simulink model "Vehicle_Model_14DOF"  (R2020a)
settings: Solver=ode23s  StartTime=0.0  StopTime=8  RelTol=1e-2  EnableMultiTasking=on
model workspace (MAT data in the model file):
  Csfl = 100
  Csfr = 100
  Csrl = 100
  Csrr = 100
  Hp = 0.35
  Ksfl = 100
  Ksfr = 100
  Ksrl = 100
  Ksrr = 100
undefined symbols (not defined in the file): sigbuilder_block
libraries: simulink_extras x6, simulink x1
(part 3 of 3)

== matlab function Vehicle_Model_14DOF/Full vehicle 14 D.O.F /Vehicle Handling model 7D.O.F /Yaw axis d,o,f /Sigma  moment Yaw axis ==
  data: A_O input; A_i input; Yaw output; Fxfl input; Fyfl input; Fxfr input; Fyfr input; Fxrl input; Fyrl input; Fxrr input; Fyrr input; Mzfl input; Mzfr input; Mzrl input; Mzrr input; wf input; wr input; a input; b input
function Yaw = fcn(A_O,A_i,Fxfl,Fyfl,Fxfr,Fyfr,Fxrl,Fyrl,Fxrr,Fyrr,Mzfl,Mzfr,Mzrl,Mzrr,wf,wr,a,b)

Yaw =(-(wf./2).*Fxfl.*cos(A_O))+((wf./2).*Fxfr.*cos(A_i))-((wr./2).*Fxrl)+((wr./2).*Fxrr)+((wf./2).*Fyfl.*sin(A_O))-((wf./2).*Fyfr.*sin(A_i))+(a.*Fxfl.*sin(A_O))+(a.*Fyfl.*cos(A_O))+(a.*Fxfr.*sin(A_i))+(a.*Fyfr.*cos(A_i))-(b.*Fyrl)-(b.*Fyrr)+(Mzfl)+(Mzfr)+(Mzrl)+(Mzrr);

== matlab function Vehicle_Model_14DOF/Full vehicle 14 D.O.F /Tiremodel/Tire front right/Fx/MATLAB Function ==
  data: ffz input; Fx output; xx input
function Fx = fcn(ffz,xx)

%xx is the slip ratio -- expressed as fraction
D=2.776
C=1.6099
B=14.3014
E=1.0224
sv=0.1221
sh=0
Fx = D.* ffz .*sin(C.* atan((B.*(xx+sh*ffz))- E*(B.* (xx+sh*ffz)- atan(B.*(xx+sh*ffz))))) ;

== matlab function Vehicle_Model_14DOF/Full vehicle 14 D.O.F /Vehicle Handling model 7D.O.F /Longtudinal axis D.O.F /MATLAB Function ==
  data: A_o input; A_i input; AX output; Fxfl input; Fyfl input; Fxfr input; Fyfr input; Fxrl input; Fxrr input; Vx input; Ro input; Ar input; Cd input
function AX = fcn(A_o,A_i,Fxfl,Fyfl,Fxfr,Fyfr,Fxrl,Fxrr, Vx, Ro, Ar, Cd)

AX = Fxfl.*cos(A_o)-Fyfl.*sin(A_o)+Fxfr.*cos(A_i)-Fyfr.*sin(A_i)+Fxrr+Fxrl - 1/2 .* Vx.^2 .* Ro .* Ar .* Cd - 70;

== matlab function Vehicle_Model_14DOF/Full vehicle 14 D.O.F /Vehicle Handling model 7D.O.F /Lateral Axis D.o.f /MATLAB Function ==
  data: A_o input; A_i input; AY output; Fyfl input; Fxfl input; Fyfr input; Fxfr input; Fyrl input; Fyrr input
function AY = fcn(A_o,A_i,Fyfl,Fxfl,Fyfr,Fxfr,Fyrl,Fyrr)

AY = Fyfl.*cos(A_o)+Fxfl.*sin(A_o)+Fyfr.*cos(A_i)+Fxfr.*sin(A_i)+Fyrl+Fyrr;

== matlab function Vehicle_Model_14DOF/Full vehicle 14 D.O.F /Vehicle Handling model 7D.O.F /Powertrain /MATLAB Function4 ==
  data: T input; Fx input; RPM input; m output; Rw input
function m = fcn(T, Fx, RPM, Rw)
if (RPM > 15100)
    m = Fx * Rw;
else
    m=T;
end
end

== matlab function Vehicle_Model_14DOF/Full vehicle 14 D.O.F /Tiremodel/Tire front left/Fx/MATLAB Function ==
  data: ffz input; Fx output; xx input
function Fx = fcn(ffz,xx)

%xx is the slip ratio -- expressed as fraction
D=2.776
C=1.6099
B=14.3014
E=1.0224
sv=0.1221
sh=0
Fx = D.* ffz .*sin(C.* atan((B.*(xx+sh*ffz))- E*(B.* (xx+sh*ffz)- atan(B.*(xx+sh*ffz))))) ;

== matlab function Vehicle_Model_14DOF/Full vehicle 14 D.O.F /Vehicle Handling model 7D.O.F /Powertrain /MATLAB Function5 ==
  data: T input; Fx input; RPM input; m output; Rw input
function m = fcn(T, Fx, RPM, Rw)
if (RPM > 15100)
    m = Fx * Rw;
else
    m=T;
end
end

== matlab function Vehicle_Model_14DOF/Full vehicle 14 D.O.F /Tiremodel/LCO width 6 psi 14/Fx/MATLAB Function ==
  data: ffz input; Fx output; xx input
function Fx = fcn(ffz,xx)

%xx is the slip ratio -- expressed as fraction
D= 12.3158
C=0.2162
B=12.9458 
E=1.0917


sv=0
sh=0
Fx = D.* ffz .*sin(C.* atan((B.*(xx+sh*ffz))- E*(B.* (xx+sh*ffz)- atan(B.*(xx+sh*ffz))))) + sv*ffz;

== matlab function Vehicle_Model_14DOF/Full vehicle 14 D.O.F /Tiremodel/Tire front left/fy/MATLAB Function ==
  data: ffz input; Fx output; xx input
function Fx = fcn(ffz,xx)

%xx is the slip ratio -- expressed as fraction
D = -2.8334
C =  1.5184
B =    0.2461
E =   0.4953


Fx = D.* ffz .*sin(C.* atan((B.*(xx))- E*(B.* (xx)- atan(B.*(xx))))) ;

== matlab function Vehicle_Model_14DOF/Full vehicle 14 D.O.F /Tiremodel/LCO width 6 psi 14/fy/MATLAB Function ==
  data: ffz input; Fx output; xx input
function Fx = fcn(ffz,xx)

%xx is the slip ratio -- expressed as fraction
D=-2.4199
C=3.6531
B=0.0586
E=3.1915





Fx = D.* ffz .*sin(C.* atan((B.*(xx))- E*(B.* (xx)- atan(B.*(xx))))) ;

== matlab function Vehicle_Model_14DOF/Full vehicle 14 D.O.F /Tiremodel/LCO width 6 psi 14/fy1/MZ/MATLAB Function ==
  data: ffz input; Fx output; xx input
function Fx = fcn(ffz,xx)

%xx is the slip ratio -- expressed as fraction
D=-14.1402
C=-0.0029
B=1.0476
E=1.1218



Fx = D.* ffz .*sin(C.* atan((B.*(xx))- E*(B.* (xx)- atan(B.*(xx))))) ;

== matlab function Vehicle_Model_14DOF/Full vehicle 14 D.O.F /Tiremodel/R25b width 7 psi 14/Fx/MATLAB Function ==
  data: ffz input; Fx output; xx input
function Fx = fcn(ffz,xx)

%xx is the slip ratio -- expressed as fraction
D=2.3835
C=1.1725
B=14.4401
E=0.1925

sv=0
sh=0
Fx = D.* ffz .*sin(C.* atan((B.*(xx+sh*ffz))- E*(B.* (xx+sh*ffz)- atan(B.*(xx+sh*ffz))))) + sv*ffz;

== matlab function Vehicle_Model_14DOF/Full vehicle 14 D.O.F /Tiremodel/R25b width 7 psi 14/fy/MATLAB Function ==
  data: ffz input; Fx output; xx input
function Fx = fcn(ffz,xx)

%xx is the slip ratio -- expressed as fraction
D= -2.5960
C= 1.6785    
B= 0.1612    
E= 1.3667



Fx = D.* ffz .*sin(C.* atan((B.*(xx))- E*(B.* (xx)- atan(B.*(xx))))) ;

== matlab function Vehicle_Model_14DOF/Full vehicle 14 D.O.F /Tiremodel/R25b width 7 psi 14/fy1/MZ/MATLAB Function ==
  data: ffz input; Fx output; xx input
function Fx = fcn(ffz,xx)

%xx is the slip ratio -- expressed as fraction
D = -0.8015
C = -0.0512
B = 0.8235
E = 1.1950



Fx = D.* ffz .*sin(C.* atan((B.*(xx))- E*(B.* (xx)- atan(B.*(xx))))) ;

== matlab function Vehicle_Model_14DOF/Full vehicle 14 D.O.F /Tiremodel/R25b width 6 psi 14/Fx/MATLAB Function ==
  data: ffz input; Fx output; xx input
function Fx = fcn(ffz,xx)

%xx is the slip ratio -- expressed as fraction
D= 2.4699    
C=0.8676   
B=15.9036    
E=0.1161

sv=0
sh=0
Fx = D.* ffz .*sin(C.* atan((B.*(xx+sh*ffz))- E*(B.* (xx+sh*ffz)- atan(B.*(xx+sh*ffz))))) + sv*ffz;

== matlab function Vehicle_Model_14DOF/Full vehicle 14 D.O.F /Tiremodel/R25b width 6 psi 14/fy/MATLAB Function ==
  data: ffz input; Fx output; xx input
function Fx = fcn(ffz,xx)

%xx is the slip ratio -- expressed as fraction
D= -2.4262 
C= 38.3467
B= 0.0066
E= 230



Fx = D.* ffz .*sin(C.* atan((B.*(xx))- E*(B.* (xx)- atan(B.*(xx))))) ;

== matlab function Vehicle_Model_14DOF/Full vehicle 14 D.O.F /Tiremodel/R25b width 6 psi 14/fy1/MZ/MATLAB Function ==
  data: ffz input; Fx output; xx input
function Fx = fcn(ffz,xx)

%xx is the slip ratio -- expressed as fraction
D = -0.8415
C = -0.0512
B = 0.8235
E = 1.1959




Fx = D.* ffz .*sin(C.* atan((B.*(xx))- E*(B.* (xx)- atan(B.*(xx))))) ;

== matlab function Vehicle_Model_14DOF/Full vehicle 14 D.O.F /Tiremodel/R25b width 7 psi 10/Fx/MATLAB Function ==
  data: ffz input; Fx output; xx input
function Fx = fcn(ffz,xx)

%xx is the slip ratio -- expressed as fraction
D=2.4969
C=1.1361
B=15.4159
E=0.3780

sv=0
sh=0
Fx = D.* ffz .*sin(C.* atan((B.*(xx+sh*ffz))- E*(B.* (xx+sh*ffz)- atan(B.*(xx+sh*ffz))))) + sv*ffz;

== matlab function Vehicle_Model_14DOF/Full vehicle 14 D.O.F /Tiremodel/R25b width 7 psi 10/fy/MATLAB Function ==
  data: ffz input; Fx output; xx input
function Fx = fcn(ffz,xx)

%xx is the slip ratio -- expressed as fraction
D= -2.7860
C= 1.6785    
B= 0.1712    
E= 1.3667



Fx = D.* ffz .*sin(C.* atan((B.*(xx))- E*(B.* (xx)- atan(B.*(xx))))) ;

== matlab function Vehicle_Model_14DOF/Full vehicle 14 D.O.F /Tiremodel/Tire front right/fy/MATLAB Function ==
  data: ffz input; Fx output; xx input
function Fx = fcn(ffz,xx)

%xx is the slip ratio -- expressed as fraction
D = -2.8334
C =  1.5184
B =    0.2461
E =   0.4953


Fx = D.* ffz .*sin(C.* atan((B.*(xx))- E*(B.* (xx)- atan(B.*(xx))))) ;

== matlab function Vehicle_Model_14DOF/Full vehicle 14 D.O.F /Tiremodel/R25b width 7 psi 10/MZ/MZ/MATLAB Function ==
  data: ffz input; Fx output; xx input
function Fx = fcn(ffz,xx)

%xx is the slip ratio -- expressed as fraction
D= -0.0473   
C= -0.8214    
B= 1.0   
E= 1.133



Fx = D.* ffz .*sin(C.* atan((B.*(xx))- E*(B.* (xx)- atan(B.*(xx))))) ;

== matlab function Vehicle_Model_14DOF/Full vehicle 14 D.O.F /Tiremodel/R25b width 6 psi 10/Fx/MATLAB Function ==
  data: ffz input; Fx output; xx input
function Fx = fcn(ffz,xx)

%xx is the slip ratio -- expressed as fraction
D=2.3207
C=1.3835
B=16.6275
E=0.5292


sv=0
sh=0
Fx = D.* ffz .*sin(C.* atan((B.*(xx+sh*ffz))- E*(B.* (xx+sh*ffz)- atan(B.*(xx+sh*ffz))))) + sv*ffz;

== matlab function Vehicle_Model_14DOF/Full vehicle 14 D.O.F /Tiremodel/R25b width 6 psi 10/fy/MATLAB Function ==
  data: ffz input; Fx output; xx input
function Fx = fcn(ffz,xx)

%xx is the slip ratio -- expressed as fraction
D= -2.6862 
C= 38.3467
B= 0.0066
E= 230



Fx = D.* ffz .*sin(C.* atan((B.*(xx))- E*(B.* (xx)- atan(B.*(xx))))) ;

== matlab function Vehicle_Model_14DOF/Full vehicle 14 D.O.F /Tiremodel/R25b width 6 psi 10/fy1/MZ/MATLAB Function ==
  data: ffz input; Fx output; xx input
function Fx = fcn(ffz,xx)

%xx is the slip ratio -- expressed as fraction
D = -0.8415
C = -0.0512
B = 0.8235
E = 1.1859




Fx = D.* ffz .*sin(C.* atan((B.*(xx))- E*(B.* (xx)- atan(B.*(xx))))) ;

== matlab function Vehicle_Model_14DOF/Full vehicle 14 D.O.F /Tiremodel/LCO width 6 psi 10/Fx/MATLAB Function ==
  data: ffz input; Fx output; xx input
function Fx = fcn(ffz,xx)

%xx is the slip ratio -- expressed as fraction
D=2.2791
C=1.7652
B=8.0954
E=0.6957

sv=0
sh=0
Fx = D.* ffz .*sin(C.* atan((B.*(xx+sh*ffz))- E*(B.* (xx+sh*ffz)- atan(B.*(xx+sh*ffz))))) + sv*ffz;

== matlab function Vehicle_Model_14DOF/Full vehicle 14 D.O.F /Tiremodel/LCO width 6 psi 10/fy/MATLAB Function ==
  data: ffz input; Fx output; xx input
function Fx = fcn(ffz,xx)

%xx is the slip ratio -- expressed as fraction
D=-2.6199
C=3.6531
B=0.0586
E=3.1915




Fx = D.* ffz .*sin(C.* atan((B.*(xx))- E*(B.* (xx)- atan(B.*(xx))))) ;

== matlab function Vehicle_Model_14DOF/Full vehicle 14 D.O.F /Tiremodel/LCO width 6 psi 10/fy1/MZ/MATLAB Function ==
  data: ffz input; Fx output; xx input
function Fx = fcn(ffz,xx)

%xx is the slip ratio -- expressed as fraction
D=-23.1402
C=-0.0029
B=0.45
E=1.3




Fx = D.* ffz .*sin(C.* atan((B.*(xx))- E*(B.* (xx)- atan(B.*(xx))))) ;

== matlab function Vehicle_Model_14DOF/Full vehicle 14 D.O.F /Tiremodel/Tire front left/fy1/MZ/MATLAB Function ==
  data: ffz input; Fx output; xx input
function Fx = fcn(ffz,xx)

%xx is the slip ratio -- expressed as fraction
D = -2.0312
C = -0.0268
B = 1.0528
E = 1.1437


Fx = D.* ffz .*sin(C.* atan((B.*(xx))- E*(B.* (xx)- atan(B.*(xx))))) ;

== matlab function Vehicle_Model_14DOF/Full vehicle 14 D.O.F /Tiremodel/Tire front right/fy1/MZ/MATLAB Function ==
  data: ffz input; Fx output; xx input
function Fx = fcn(ffz,xx)

%xx is the slip ratio -- expressed as fraction
D = -2.0312
C = -0.0268
B = 1.0528
E = 1.1437


Fx = D.* ffz .*sin(C.* atan((B.*(xx))- E*(B.* (xx)- atan(B.*(xx))))) ;

== matlab function Vehicle_Model_14DOF/Full vehicle 14 D.O.F /Tiremodel/Tire rear left/Fx/MATLAB Function ==
  data: ffz input; Fx output; xx input
function Fx = fcn(ffz,xx)

%xx is the slip ratio -- expressed as fraction
D=2.776
C=1.6099
B=14.3014
E=1.0224
sv=0.1221
sh=0
Fx = D.* ffz .*sin(C.* atan((B.*(xx+sh*ffz))- E*(B.* (xx+sh*ffz)- atan(B.*(xx+sh*ffz))))) ;

== matlab function Vehicle_Model_14DOF/Full vehicle 14 D.O.F /Tiremodel/Tire rear left/fy/MATLAB Function ==
  data: ffz input; Fx output; xx input
function Fx = fcn(ffz,xx)

%xx is the slip ratio -- expressed as fraction
D = -2.8334
C =  1.5184
B =    0.2461
E =   0.4953


Fx = D.* ffz .*sin(C.* atan((B.*(xx))- E*(B.* (xx)- atan(B.*(xx))))) ;

== matlab function Vehicle_Model_14DOF/Full vehicle 14 D.O.F /Tiremodel/Tire rear left/fy1/MZ/MATLAB Function ==
  data: ffz input; Fx output; xx input
function Fx = fcn(ffz,xx)

%xx is the slip ratio -- expressed as fraction
D = -2.0312
C = -0.0268
B = 1.0528
E = 1.1437


Fx = D.* ffz .*sin(C.* atan((B.*(xx))- E*(B.* (xx)- atan(B.*(xx))))) ;

== matlab function Vehicle_Model_14DOF/Full vehicle 14 D.O.F /Tiremodel/Tire rear Right/Fx/MATLAB Function ==
  data: ffz input; Fx output; xx input
function Fx = fcn(ffz,xx)

%xx is the slip ratio -- expressed as fraction
D=2.776
C=1.6099
B=14.3014
E=1.0224
sv=0.1221
sh=0
Fx = D.* ffz .*sin(C.* atan((B.*(xx+sh*ffz))- E*(B.* (xx+sh*ffz)- atan(B.*(xx+sh*ffz))))) ;

== matlab function Vehicle_Model_14DOF/Full vehicle 14 D.O.F /Tiremodel/Tire rear Right/fy/MATLAB Function ==
  data: ffz input; Fx output; xx input
function Fx = fcn(ffz,xx)

%xx is the slip ratio -- expressed as fraction
D = -2.8334
C =  1.5184
B =    0.2461
E =   0.4953


Fx = D.* ffz .*sin(C.* atan((B.*(xx))- E*(B.* (xx)- atan(B.*(xx))))) ;
